simulink model "camdec"  (R2023b)
settings: Solver=FixedStepAuto  StartTime=0.0  StopTime=inf  RelTol=1e-3
libraries: speedgoatlib_IO133 x3, eePwmGenerator x1, slrealtimeiplib x1
settings Model: Creator=abhin  LastModifiedBy=abhin
settings SolverCC: ConcurrentTasks=on  PositivePriorityOrder=on
settings OptimizationCC: BlockReduction=off  OptimizeBlockIOStorage=off
settings DebuggingCC: TasksWithSamePriorityMsg=none
settings HardwareCC: ProdBitPerLong=64  ProdLongLongMode=on  ProdHWDeviceType=Intel->x86-64 (Linux 64)
settings RTWCC: Description=Simulink Real-Time  SystemTargetFile=slrealtime.tlc  TemplateMakefile=slrealtime_default_tmf  Toolchain=Simulink Real-Time Toolchain  BuildConfiguration=Faster Runs  CodeExecutionProfiling=on  TargetLang=C++

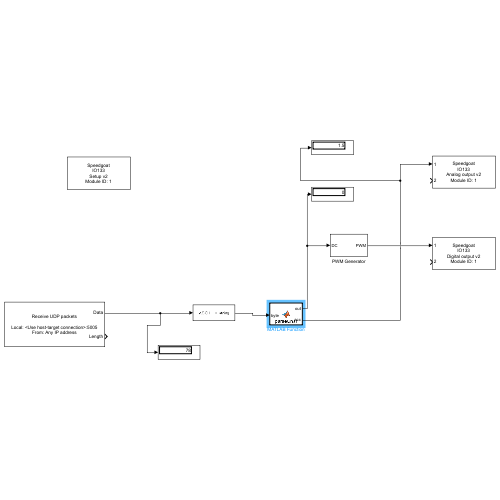
[thumbnail: Simulink's stored preview of the top-level diagram]
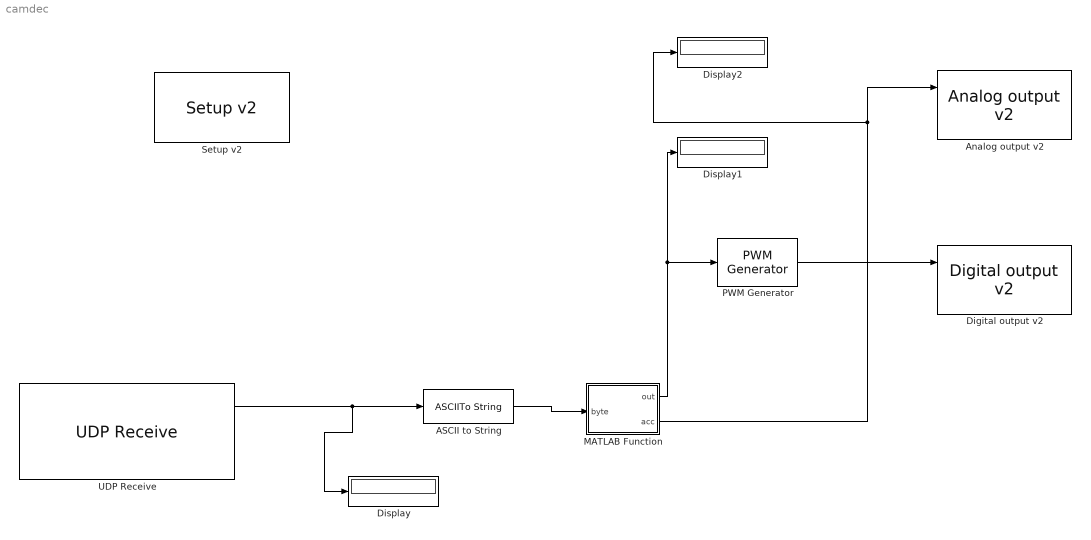
== system camdec ==
  ASCII to String : ASCIIToString
  "Analog output v2 " : speedgoatlib_IO133/Analog output v2   parModuleId=1  parSampleTime=5e-5  parPciSlot=-1  parDacChannels=[1 2]  parDacVoltageRange=[1 1 1 1 1 1 1 1]  parDacInitValues=[0 0]  parDacReset=[1 1]  parDacSyncOut=1  parDacDmaEnable=0  parDacActiveDmaDevices=[1 1]  parDacDmaLatency=2  parDacFrameSize=100
      settings: SourceProductName=Simulink Real-Time: Speedgoat I/O Blockset
  "Digital output v2 " : speedgoatlib_IO133/Digital output v2   parModuleId=1  parSampleTime=5e-5  parPciSlot=-1  parDoChannels=[1 2]  parDoInitValues=[0 0]  parDoReset=[1 1]
      settings: SourceProductName=Simulink Real-Time: Speedgoat I/O Blockset
  Display : Display
  Display1 : Display
  Display2 : Display
  MATLAB Function : MATLAB Function  TreatAsAtomicUnit=on
  PWM Generator : eePwmGenerator/PWM Generator  CarrCount=Up  Tper=0.001  Tdelay=0  Ts=5e-5
  "Setup v2 " : speedgoatlib_IO133/Setup v2   parPciSlot=-1  parModuleId=1  parInterModuleSync=None  parConvClockBaseRate=20MHz  parConvClock1Divider=20000  parConvClock2Divider=20000  parFrameTriggerEnable=off  parFrameTriggerDivider=10  parConvClock1BaseRate=1  parConvClock2BaseRate=1  parFrameTriggerClock=1  parAdcChannels=[1 2]  parAdcRange1=+-5V  parAdcRange2=+-5V  parAdcVoltageRange=[1 1]  parAdcOversampling1=None  parAdcOversampling2=None  parAdcOversamplRate=[1 1]  parAdcAutoCorrection=on  parAdcContSampling=off  parAdcDmaEnable=off  parAdcDmaClock=Clock 1  parAdcFrameSize_=100  parAdcSampleTime_=-1  parAdcActiveDmaDevices=[1 1]  parAdcFrameTriggerEnable=0  parAdcFrameSize=100  parAdcSampleTime=0.1  parDacChannels=[1 2]  parDacInitValues=0  parDacReset=1  parDacRange1=0-5V  parDacRange2=0-5V  parDacRange3=0-5V  parDacRange4=0-5V  parDacRange5=0-5V  parDacRange6=0-5V  parDacRange7=0-5V  parDacRange8=0-5V  parDacVoltageRange=[1 1 1 1 1 1 1 1]  parDacAutoCorrection=on  parDacSyncOut=on  parDacDmaEnable=off  parDacDmaLatency=Until next frame  parDacDmaClock=Clock 1  parDacFrameSize_=100  parDacSampleTime_=-1  parDacActiveDmaDevices=[1 1]  parDacFrameTriggerEnable=0  parDacFrameSize=100  parDacSampleTime=0.1  parDoChannels=[1 2]  parDoInitValues=0  parDoReset=1  parDiChannels=[3 4]  parDiDebounceEnable=off  parDiDebounceTime=0  parDiDebounceValue=0  parDioPullRefFront=Pull-up 3.3V  parDioPullRefRear=Floating
      settings: SourceProductName=Simulink Real-Time: Speedgoat I/O Blockset
  UDP Receive : slrealtimeiplib/UDP Receive  useHostTargetConn=on  ipAddress=10.10.10.15  localPort=5005  rcvWidth=1  rcvFmAny=on  fmAddress='10.10.10.10'  sampleTime=-1  enableMessage=off  maxPackets=1
  wires:
  PWM Generator/1 -> "Digital output v2 "/1
  MATLAB Function/1(out) -> Display1/1, PWM Generator/1
  UDP Receive/1 -> Display/1, ASCII to String/1
  ASCII to String/1 -> MATLAB Function/1(byte)
  MATLAB Function/2(acc) -> Display2/1, "Analog output v2 "/1

== matlab function camdec/MATLAB Function ==
  data: byte input; out output; acc output
function [out,acc] = parseChar(byte)

    if byte == "Y"
        out = 1;
        acc = 0;
    else
        out = 0;
        acc = 1.5;
    end
end
